simulink model "rePark"  (R2022b)
settings: Solver=VariableStepAuto  StartTime=0.0  StopTime=10.0  RelTol=1e-3
settings Model: Creator=15403  LastModifiedBy=15403

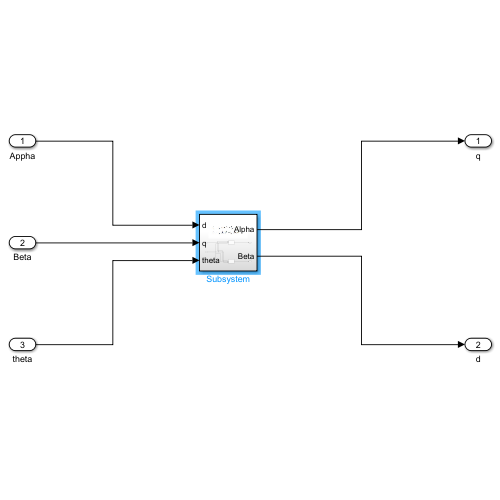
[thumbnail: Simulink's stored preview of the top-level diagram]
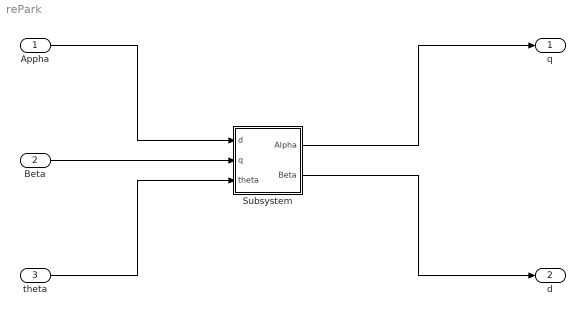
== system rePark ==
  Appha : Inport
  Beta : Inport  Port=2
  theta : Inport  Port=3
  Subsystem : Subsystem
  q : Outport
  d : Outport  Port=2
  wires:
  Subsystem/1(Alpha) -> q/1
  theta/1 -> Subsystem/3(theta)
  Appha/1 -> Subsystem/1(d)
  Beta/1 -> Subsystem/2(q)
  Subsystem/2(Beta) -> d/1

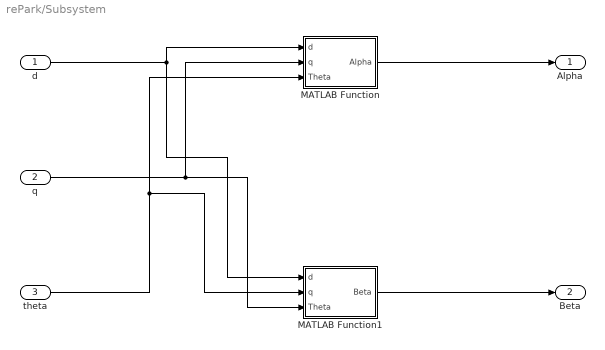
== system rePark/Subsystem ==
  d : Inport
  q : Inport  Port=2
  theta : Inport  Port=3
  MATLAB Function : MATLAB Function  TreatAsAtomicUnit=on
  MATLAB Function1 : MATLAB Function  TreatAsAtomicUnit=on
  Alpha : Outport
  Beta : Outport  Port=2
  wires:
  theta/1 -> MATLAB Function1/2(q), MATLAB Function/3(Theta)
  MATLAB Function1/1(Beta) -> Beta/1
  q/1 -> MATLAB Function1/3(Theta), MATLAB Function/2(q)
  d/1 -> MATLAB Function1/1(d), MATLAB Function/1(d)
  MATLAB Function/1(Alpha) -> Alpha/1

== matlab function rePark/Subsystem/MATLAB Function ==
  data: d input; Alpha output; q input; Theta input
function Alpha = fcn(d, q, Theta)

Alpha = q * cosd(Theta) + d * sind(Theta);

== matlab function rePark/Subsystem/MATLAB Function1 ==
  data: d input; Beta output; q input; Theta input
function Beta = fcn(d, q, Theta)

Beta = -q * sind(Theta) + d * cosd(Theta);
